simulink model "FMsendrec"  (Simulink 9.0)
settings: Solver=FixedStepDiscrete  StartTime=0.0  StopTime=inf  RelTol=1e-3
PreLoadFcn:
  | setenv('MW_MINGW64_LOC','C:\TDM-GCC-64')
StartFcn:
  | tic
StopFcn:
  | toc;
undefined symbols (not defined in the file): magnitude
libraries: UN_HIL_Lib x4, dspobslib x2, dsparch4 x1
Description:
  | QPSK Transmitter and Receiver.
  | 
  | This model shows the implementation of a QPSK transmitter and receiver.
settings Model: FPTRunName=Active  Creator=The MathWorks Inc.  LastModifiedBy=minel
settings DataIOCC: LimitDataPoints=on  SignalLoggingSaveFormat=ModelDataLogs  SaveOutput=off  SaveTime=off
settings OptimizationCC: BooleanDataType=off  DefaultParameterBehavior=Inlined  ExpressionDepthLimit=2147483647  LocalBlockOutputs=off
settings DebuggingCC: AlgebraicLoopMsg=error  SolverPrmCheckMsg=warning  SingleTaskRateTransMsg=error  ParameterPrecisionLossMsg=none  FcnCallInpInsideContextMsg=warning  StateNameClashWarn=warning
settings HardwareCC: TargetBitPerPointer=64  TargetBitPerSizeT=64  TargetBitPerPtrDiffT=64  TargetLongLongMode=on  TargetIntDivRoundTo=Zero  TargetEndianess=LittleEndian  TargetWordSize=64  TargetHWDeviceType=Generic->MATLAB Host Computer  ProdEqTarget=off
settings GRTTargetCC: GeneratePreprocessorConditionals=Disable all
settings ConfigComp: CovSFcnEnable=off
settings SimEventsCC: propDiagStatOutput=1  propPreventDuplicateEvents=0

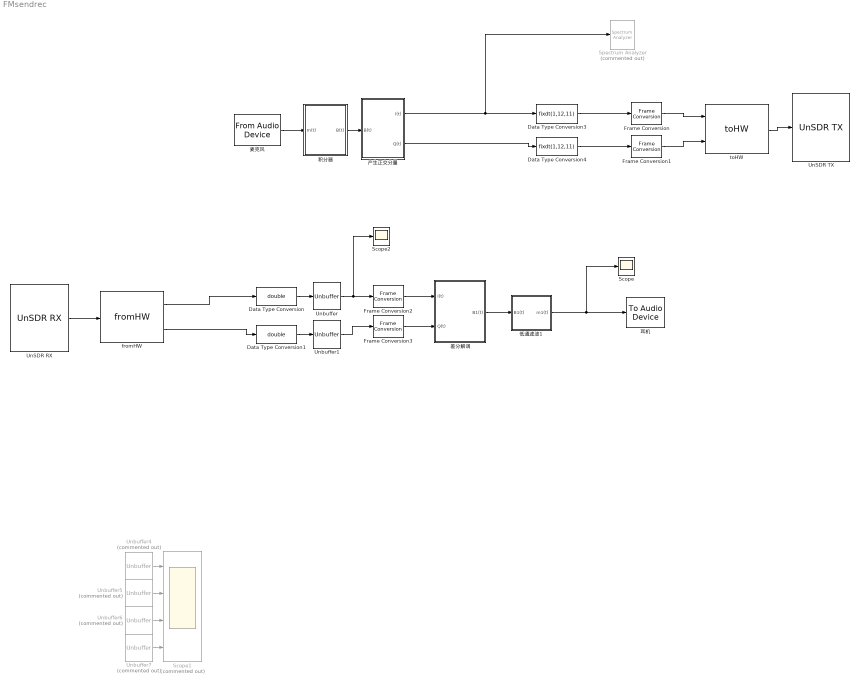
== system FMsendrec ==
  Data Type Conversion : DataTypeConversion  OutDataTypeStr=double
  Data Type Conversion1 : DataTypeConversion  OutDataTypeStr=double
  Data Type Conversion3 : DataTypeConversion  OutDataTypeStr=fixdt(1,12,11)
  Data Type Conversion4 : DataTypeConversion  OutDataTypeStr=fixdt(1,12,11)
  Frame Conversion{,1..3} (4 alike) : FrameConversion  InheritSamplingMode=off  OutFrame=Sample-based
  Scope : Scope
  Scope1 : Scope  Commented=on  NumInputPorts=4
  Scope2 : Scope
  Spectrum Analyzer : SpectrumAnalyzer  Commented=on
  UnSDR RX : UN_HIL_Lib/UnSDR RX  SystemSampleTime=-1
      settings: SourceProductName=HIL Blockset
  UnSDR TX : UN_HIL_Lib/UnSDR TX  SystemSampleTime=-1
      settings: SourceProductName=HIL Blockset
  Unbuffer : Unbuffer
  Unbuffer1 : Unbuffer
  Unbuffer{4..7} (4 alike) : Unbuffer  Commented=on
  fromHW : UN_HIL_Lib/fromHW  sp=1/48e3
      settings: SourceProductName=HIL Blockset
  toHW : UN_HIL_Lib/toHW  SystemSampleTime=-1
      settings: SourceProductName=HIL Blockset
  产生正交分量 : Subsystem
  低通滤波1 : Subsystem
  差分解调 : Subsystem
  积分器 : Subsystem
  耳机 : dspobslib/To Audio Device  deviceName=扬声器/听筒 (Realtek Audio)  inheritSampleRate=on  sampleRate=44100  deviceDatatype=Determine from input data type  autoBufferSize=on  bufferSize=4096  queueDuration=2  defaultOutputChannelMapping=on  outputChannelMapping=1:2  outputNumUnderrunSamples=off
      settings: SourceProductName=DSP System Toolbox  SourceProductBaseCode=DS
  麦克风 : dspobslib/From Audio Device  deviceName=麦克风 (Realtek Audio)  numChannels=1  sampleRate=48000  deviceDatatype=Determine from output data type  autoBufferSize=on  bufferSize=4096  queueDuration=1.0  frameSize=1  outputDatatype=single  defaultInputChannelMapping=on  inputChannelMapping=1:2  outputNumOverrunSamples=off  OutputFrames=on
      settings: SourceProductName=DSP System Toolbox  SourceProductBaseCode=DS
  wires:
  Unbuffer5/1 -> Scope1/2
  Unbuffer6/1 -> Scope1/3
  Unbuffer7/1 -> Scope1/4
  Unbuffer4/1 -> Scope1/1
  Data Type Conversion3/1 -> Frame Conversion/1
  Data Type Conversion4/1 -> Frame Conversion1/1
  Frame Conversion1/1 -> toHW/2
  Frame Conversion/1 -> toHW/1
  Unbuffer/1 -> Scope2/1, Frame Conversion2/1
  fromHW/1 -> Data Type Conversion/1
  Data Type Conversion/1 -> Unbuffer/1
  fromHW/2 -> Data Type Conversion1/1
  麦克风/1 -> 积分器/1(m(t))
  积分器/1(B(t)) -> 产生正交分量/1(B(t))
  低通滤波1/1(m1(t)) -> Scope/1, 耳机/1
  差分解调/1(B1(t)) -> 低通滤波1/1(B1(t))
  Data Type Conversion1/1 -> Unbuffer1/1
  Unbuffer1/1 -> Frame Conversion3/1
  产生正交分量/1(I(t)) -> Data Type Conversion3/1, Spectrum Analyzer/1
  产生正交分量/2(Q(t)) -> Data Type Conversion4/1
  Frame Conversion2/1 -> 差分解调/1(I(t))
  Frame Conversion3/1 -> 差分解调/2(Q(t))
  toHW/1 -> UnSDR TX/1
  UnSDR RX/1 -> fromHW/1

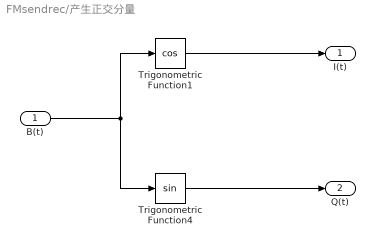
== system FMsendrec/产生正交分量 ==
  B(t) : Inport
  Trigonometric Function1 : Trigonometry  Operator=cos  NumberOfIterations=16
  Trigonometric Function4 : Trigonometry  NumberOfIterations=16
  I(t) : Outport
  Q(t) : Outport  Port=2
  wires:
  Trigonometric Function1/1 -> I(t)/1
  B(t)/1 -> Trigonometric Function4/1, Trigonometric Function1/1
  Trigonometric Function4/1 -> Q(t)/1

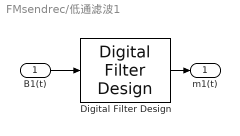
== system FMsendrec/低通滤波1 ==
  B1(t) : Inport
  Digital Filter Design : dsparch4/Digital Filter Design  mwdsp_browser_bugfix_var=off
  m1(t) : Outport
  wires:
  B1(t)/1 -> Digital Filter Design/1
  Digital Filter Design/1 -> m1(t)/1

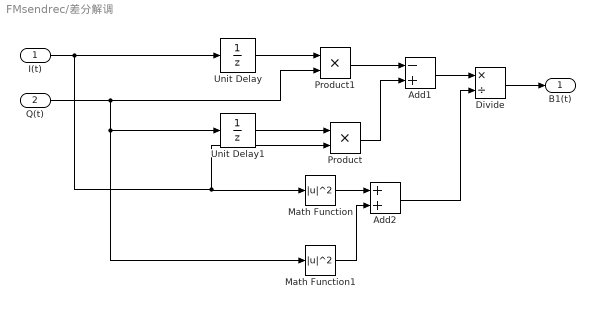
== system FMsendrec/差分解调 ==
  I(t) : Inport
  Q(t) : Inport  Port=2
  Add1 : Sum  Inputs=-+
  Add2 : Sum
  Divide : Product  Inputs=*/
  Math Function : Math  Operator=magnitude^2  SaturateOnIntegerOverflow=on
  Math Function1 : Math  Operator=magnitude^2  SaturateOnIntegerOverflow=on
  Product : Product  RndMeth=Zero
  Product1 : Product  RndMeth=Zero
  Unit Delay : UnitDelay  SampleTime=-1
  Unit Delay1 : UnitDelay  SampleTime=-1
  B1(t) : Outport
  wires:
  Add1/1 -> Divide/1
  Add2/1 -> Divide/2
  Product/1 -> Add1/2
  Product1/1 -> Add1/1
  Unit Delay/1 -> Product1/1
  Unit Delay1/1 -> Product/1
  Q(t)/1 -> Math Function1/1, Unit Delay1/1, Product1/2
  I(t)/1 -> Product/2, Math Function/1, Unit Delay/1
  Math Function/1 -> Add2/1
  Math Function1/1 -> Add2/2
  Divide/1 -> B1(t)/1

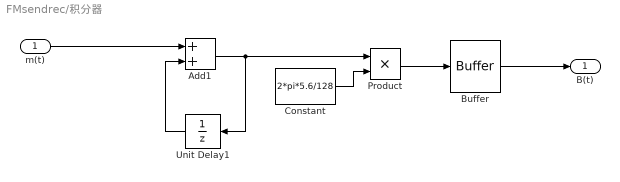
== system FMsendrec/积分器 ==
  m(t) : Inport
  Add1 : Sum  OutDataTypeStr=Inherit: Same as first input
  Buffer : Buffer  N=4096
  Constant : Constant  Value=2*pi*5.6/128  VectorParams1D=off  SampleTime=-1
  Product : Product  RndMeth=Zero  OutDataTypeStr=Inherit: Same as first input
  Unit Delay1 : UnitDelay  SampleTime=-1
  B(t) : Outport
  wires:
  Product/1 -> Buffer/1
  Constant/1 -> Product/2
  Add1/1 -> Product/1, Unit Delay1/1
  Unit Delay1/1 -> Add1/2
  m(t)/1 -> Add1/1
  Buffer/1 -> B(t)/1
